simulink model "SysStateMachine"  (R2016b)
settings: Solver=FixedStepAuto  StartTime=0.0  StopTime=inf  RelTol=1e-3
undefined symbols (not defined in the file or in its folder): Chart, nav_statemachine_lib, paramInit
settings Model: Creator=chenjianhui  LastModifiedBy=chenjh43
settings OptimizationCC: MaxStackSize=64
settings DebuggingCC: ParameterTunabilityLossMsg=error
settings HardwareCC: ProdBitPerLong=64  ProdHWDeviceType=Intel->x86-64 (Linux 64)
settings RTWCC: SystemTargetFile=ert.tlc  HardwareBoard=Robot Operating System (ROS)  TLCOptions="-aInlineSetEventsForThisBaseRateFcn=TLC_FALSE -aSuppressMultiTaskScheduler=TLC_FALSE  -aRateBasedStepFcn=0"  TemplateMakefile=ert_default_tmf  Description=Embedded Coder  GenerateReport=on  Toolchain=Catkin  IncludeHyperlinkInReport=on  LaunchReport=on  TargetLang=C++  GenerateTraceInfo=on  GenerateTraceReport=on  GenerateTraceReportSl=on  GenerateTraceReportSf=on  GenerateTraceReportEml=on  GenerateWebview=on
settings CodeAppCC: ForceParamTrailComments=on  IgnoreCustomStorageClasses=off  OperatorAnnotations=on  SimulinkDataObjDesc=on  SFDataObjDesc=on  MATLABFcnDesc=on  InsertBlockDesc=on  MATLABSourceComments=on

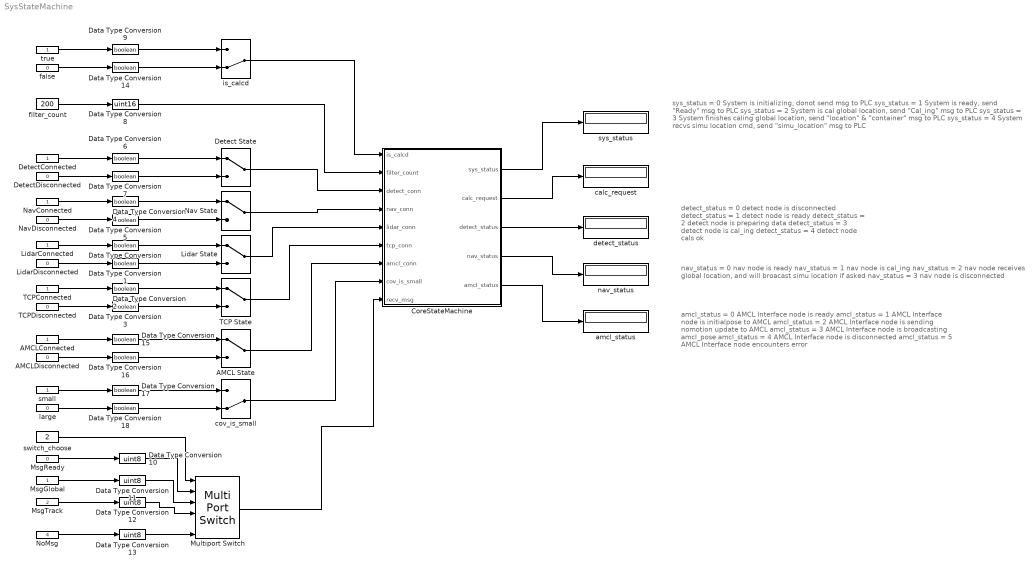
== system SysStateMachine ==
  note: sys_status = 0	System is initializing, donot send msg to PLC
      | sys_status = 1	System is ready, send "Ready" msg to PLC
      | sys_status = 2	System is cal global location, send "Cal_ing" msg to PLC
      | sys_status = 3	System finishes caling global location, send "location" & "container" msg to PLC
      | sys_status = 4	System recvs simu location cmd, send "simu_location" msg to PLC
  note: nav_status = 0 		nav node is ready
      | nav_status = 1 		nav node is cal_ing
      | nav_status = 2 		nav node receives global location, and will broacast simu location if asked
      | nav_status = 3		nav node is disconnected
  note: amcl_status = 0 AMCL Interface node is ready
      | amcl_status = 1 AMCL Interface node is initialpose to AMCL
      | amcl_status = 2 AMCL Interface node is sending nomotion update to AMCL
      | amcl_status = 3 AMCL Interface node is broadcasting amcl_pose
      | amcl_status = 4 AMCL Interface node is disconnected
      | amcl_status = 5 AMCL Interface node encounters error
  note: detect_status = 0		detect node is disconnected
      | detect_status = 1 		detect node is ready
      | detect_status = 2		detect node is preparing data
      | detect_status = 3 		detect node is cal_ing
      | detect_status = 4 		detect node cals ok
  AMCL State : ManualSwitch
  AMCLConnected : Constant
  AMCLDisconnected : Constant  Value=0
  CoreStateMachine : Subsystem  InitFcn=paramInit;
  Data Type Conversion{,1..7,9,14..18} (14 alike) : DataTypeConversion  OutDataTypeStr=boolean
  Data Type Conversion{10..13} (4 alike) : DataTypeConversion  OutDataTypeStr=uint8
  Data Type Conversion8 : DataTypeConversion  OutDataTypeStr=uint16
  Detect State : ManualSwitch
  DetectConnected : Constant
  DetectDisconnected : Constant  Value=0
  Lidar State : ManualSwitch
  LidarConnected : Constant
  LidarDisconnected : Constant  Value=0
  MsgGlobal : Constant
  MsgReady : Constant  Value=0
  MsgTrack : Constant  Value=2
  Multiport Switch : MultiPortSwitch  DataPortOrder=Zero-based contiguous  Inputs=5
  Nav State : ManualSwitch
  NavConnected : Constant
  NavDisconnected : Constant  Value=0
  NoMsg : Constant  Value=4
  TCP State : ManualSwitch
  TCPConnected : Constant
  TCPDisconnected : Constant  Value=0
  amcl_status : Display
  calc_request : Display
  cov_is_small : ManualSwitch  CurrentSetting=0
  detect_status : Display
  false : Constant  Value=0
  filter_count : Constant  Value=200
  is_calcd : ManualSwitch  CurrentSetting=0
  large : Constant  Value=0
  nav_status : Display
  small : Constant
  switch_choose : Constant  Value=2
  sys_status : Display
  true : Constant
  wires:
  LidarConnected/1 -> Data Type Conversion/1
  LidarDisconnected/1 -> Data Type Conversion1/1
  TCPConnected/1 -> Data Type Conversion2/1
  TCPDisconnected/1 -> Data Type Conversion3/1
  Data Type Conversion/1 -> Lidar State/1
  Data Type Conversion1/1 -> Lidar State/2
  Data Type Conversion2/1 -> TCP State/1
  Data Type Conversion3/1 -> TCP State/2
  CoreStateMachine/1(sys_status) -> sys_status/1
  CoreStateMachine/2(calc_request) -> calc_request/1
  CoreStateMachine/3(detect_status) -> detect_status/1
  CoreStateMachine/4(nav_status) -> nav_status/1
  MsgGlobal/1 -> Data Type Conversion11/1
  MsgTrack/1 -> Data Type Conversion12/1
  Data Type Conversion11/1 -> Multiport Switch/3
  Data Type Conversion12/1 -> Multiport Switch/4
  Lidar State/1 -> CoreStateMachine/5(lidar_conn)
  TCP State/1 -> CoreStateMachine/6(tcp_conn)
  NavConnected/1 -> Data Type Conversion4/1
  NavDisconnected/1 -> Data Type Conversion5/1
  Data Type Conversion4/1 -> Nav State/1
  Data Type Conversion5/1 -> Nav State/2
  Nav State/1 -> CoreStateMachine/4(nav_conn)
  DetectConnected/1 -> Data Type Conversion6/1
  DetectDisconnected/1 -> Data Type Conversion7/1
  Data Type Conversion6/1 -> Detect State/1
  Data Type Conversion7/1 -> Detect State/2
  Detect State/1 -> CoreStateMachine/3(detect_conn)
  Data Type Conversion8/1 -> CoreStateMachine/2(filter_count)
  filter_count/1 -> Data Type Conversion8/1
  MsgReady/1 -> Data Type Conversion10/1
  NoMsg/1 -> Data Type Conversion13/1
  Data Type Conversion10/1 -> Multiport Switch/2
  true/1 -> Data Type Conversion9/1
  false/1 -> Data Type Conversion14/1
  Data Type Conversion9/1 -> is_calcd/1
  Data Type Conversion14/1 -> is_calcd/2
  is_calcd/1 -> CoreStateMachine/1(is_calcd)
  CoreStateMachine/5(amcl_status) -> amcl_status/1
  switch_choose/1 -> Multiport Switch/1
  Data Type Conversion13/1 -> Multiport Switch/6
  Multiport Switch/1 -> CoreStateMachine/9(recv_msg)
  AMCLDisconnected/1 -> Data Type Conversion16/1
  Data Type Conversion16/1 -> AMCL State/2
  AMCL State/1 -> CoreStateMachine/7(amcl_conn)
  large/1 -> Data Type Conversion18/1
  Data Type Conversion18/1 -> cov_is_small/2
  cov_is_small/1 -> CoreStateMachine/8(cov_is_small)
  Data Type Conversion17/1 -> cov_is_small/1
  small/1 -> Data Type Conversion17/1
  AMCLConnected/1 -> Data Type Conversion15/1
  Data Type Conversion15/1 -> AMCL State/1

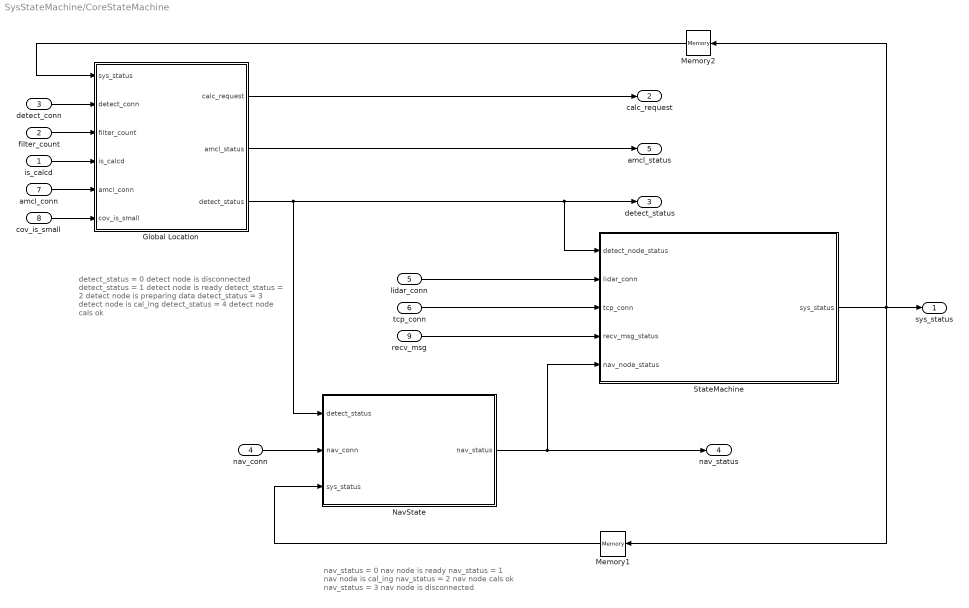
== system SysStateMachine/CoreStateMachine ==
  note: nav_status = 0 		nav node is ready
      | nav_status = 1 		nav node is cal_ing
      | nav_status = 2 		nav node cals ok
      | nav_status = 3		nav node is disconnected
  note: detect_status = 0		detect node is disconnected
      | detect_status = 1 		detect node is ready
      | detect_status = 2		detect node is preparing data
      | detect_status = 3 		detect node is cal_ing
      | detect_status = 4 		detect node cals ok
  is_calcd : Inport
  filter_count : Inport  Port=2
  detect_conn : Inport  Port=3
  nav_conn : Inport  Port=4
  lidar_conn : Inport  Port=5
  tcp_conn : Inport  Port=6
  amcl_conn : Inport  Port=7
  cov_is_small : Inport  Port=8
  recv_msg : Inport  Port=9
  Global Location : Subsystem
  Memory1 : Memory
  Memory2 : Memory
  NavState : Stateflow chart  TreatAsAtomicUnit=on
  StateMachine : Stateflow chart  AncestorBlock=nav_statemachine_lib/Chart  TreatAsAtomicUnit=on
  sys_status : Outport
  calc_request : Outport  Port=2
  detect_status : Outport  Port=3
  nav_status : Outport  Port=4
  amcl_status : Outport  Port=5
  wires:
  NavState/1(nav_status) -> nav_status/1, StateMachine/5(nav_node_status)
  StateMachine/1(sys_status) -> sys_status/1, Memory1/1, Memory2/1
  Memory1/1 -> NavState/3(sys_status)
  recv_msg/1 -> StateMachine/4(recv_msg_status)
  lidar_conn/1 -> StateMachine/2(lidar_conn)
  tcp_conn/1 -> StateMachine/3(tcp_conn)
  nav_conn/1 -> NavState/2(nav_conn)
  Global Location/3(detect_status) -> detect_status/1, StateMachine/1(detect_node_status), NavState/1(detect_status)
  Memory2/1 -> Global Location/1(sys_status)
  detect_conn/1 -> Global Location/2(detect_conn)
  filter_count/1 -> Global Location/3(filter_count)
  is_calcd/1 -> Global Location/4(is_calcd)
  amcl_conn/1 -> Global Location/5(amcl_conn)
  cov_is_small/1 -> Global Location/6(cov_is_small)
  Global Location/1(calc_request) -> calc_request/1
  Global Location/2(amcl_status) -> amcl_status/1

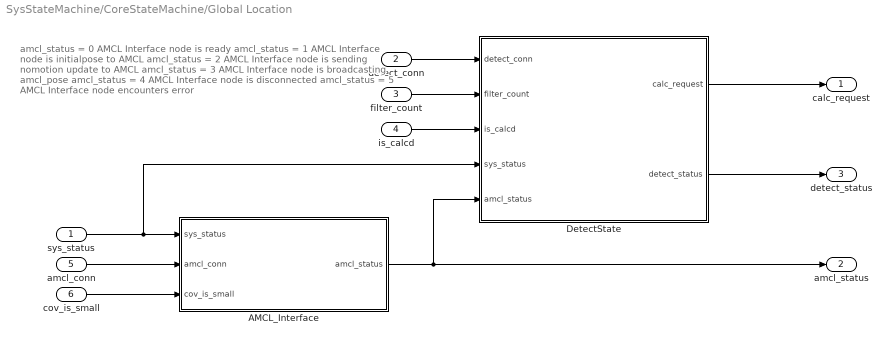
== system SysStateMachine/CoreStateMachine/Global Location ==
  note: amcl_status = 0 AMCL Interface node is ready
      | amcl_status = 1 AMCL Interface node is initialpose to AMCL
      | amcl_status = 2 AMCL Interface node is sending nomotion update to AMCL
      | amcl_status = 3 AMCL Interface node is broadcasting amcl_pose
      | amcl_status = 4 AMCL Interface node is disconnected
      | amcl_status = 5 AMCL Interface node encounters error
  sys_status : Inport
  detect_conn : Inport  Port=2
  filter_count : Inport  Port=3
  is_calcd : Inport  Port=4
  amcl_conn : Inport  Port=5
  cov_is_small : Inport  Port=6
  AMCL_Interface : Stateflow chart  TreatAsAtomicUnit=on
  DetectState : Stateflow chart  TreatAsAtomicUnit=on
  calc_request : Outport
  amcl_status : Outport  Port=2
  detect_status : Outport  Port=3
  wires:
  AMCL_Interface/1(amcl_status) -> amcl_status/1, DetectState/5(amcl_status)
  sys_status/1 -> DetectState/4(sys_status), AMCL_Interface/1(sys_status)
  DetectState/1(calc_request) -> calc_request/1
  DetectState/2(detect_status) -> detect_status/1
  detect_conn/1 -> DetectState/1(detect_conn)
  filter_count/1 -> DetectState/2(filter_count)
  is_calcd/1 -> DetectState/3(is_calcd)
  amcl_conn/1 -> AMCL_Interface/2(amcl_conn)
  cov_is_small/1 -> AMCL_Interface/3(cov_is_small)

== stateflow chart SysStateMachine/CoreStateMachine/StateMachine ==
  settings: updateMethod=DISCRETE  sampleTime=0.01
  state PCReady
    sys_status = 1;
  state Initialization
    sys_status = 0;
  state PLCReady
    sys_status = 1;
  state GlobalLocationOn
    sys_status = 2;
  state GlobalLocationOK
    sys_status = 3;
  state SimuLocation
    sys_status = 4;
  (default) -> Initialization
  Initialization -> PCReady : [lidar_conn == 1 && ...
      | tcp_conn == 1 && ...
      | detect_node_status == 1 && ...
      | nav_node_status == 0]
  SimuLocation -> Initialization [order 1] : [lidar_conn == 0 || ...
      | tcp_conn == 0 || ...
      | detect_node_status == 0 || ...
      | nav_node_status == 3]
  PCReady -> PLCReady [order 2] : [recv_msg_status == 0]
  PCReady -> Initialization [order 1] : [lidar_conn == 0 || ...
      | tcp_conn == 0 || ...
      | detect_node_status == 0 || ...
      | nav_node_status == 3]
  GlobalLocationOK -> Initialization [order 1] : [lidar_conn == 0 || ...
      | tcp_conn == 0 || ...
      | detect_node_status == 0 || ...
      | nav_node_status == 3]
  PLCReady -> Initialization [order 1] : [lidar_conn == 0 || ...
      | tcp_conn == 0 || ...
      | detect_node_status == 0 || ...
      | nav_node_status == 3]
  PLCReady -> GlobalLocationOn [order 2] : [detect_node_status == 1 && ...
      | nav_node_status == 0 && ...
      | recv_msg_status == 1]
  GlobalLocationOn -> Initialization [order 1] : [lidar_conn == 0 || ...
      | tcp_conn == 0 || ...
      | detect_node_status == 0 || ...
      | nav_node_status == 3]
  GlobalLocationOn -> GlobalLocationOK [order 2] : [detect_node_status == 4]
  SimuLocation -> GlobalLocationOn [order 2] : [recv_msg_status == 1]
  GlobalLocationOK -> SimuLocation [order 2] : [nav_node_status == 2 && ...
      | recv_msg_status == 2]
  data: detect_node_status input uint8; lidar_conn input boolean; tcp_conn input boolean; recv_msg_status input uint8; nav_node_status input uint8; sys_status output uint8

== stateflow chart SysStateMachine/CoreStateMachine/NavState ==
  settings: updateMethod=DISCRETE  sampleTime=0.01
  state NavReady
    during:nav_status = 0;
  state NavCalib
    during:nav_status = 1;
  state NavDisconn
    nav_status = 3;
  state NavOK
    during:nav_status = 2;
  NavReady -> NavCalib [order 2] : [sys_status == 2]
  NavCalib -> NavReady [order 2] : [sys_status ~= 2]
  NavCalib -> NavDisconn [order 1] : [nav_conn == 0]
  NavCalib -> NavOK [order 3] : [detect_status == 2]
  NavOK -> NavCalib [order 3] : [sys_status == 2 && ...
      | detect_status != 2]
  NavOK -> NavReady [order 2] : [sys_status == 0 || ...
      | sys_status == 1]
  NavReady -> NavDisconn [order 1] : [nav_conn == 0]
  NavDisconn -> NavReady : [nav_conn == 1]
  (default) -> NavDisconn
  NavOK -> NavDisconn [order 1] : [nav_conn == 0]
  data: detect_status input uint8; nav_conn input boolean; nav_status output uint8; sys_status input uint8

== stateflow chart SysStateMachine/CoreStateMachine/Global Location/DetectState ==
  settings: updateMethod=DISCRETE  sampleTime=0.01
  state DataPreparation
    entry:cal_count = filter_count+counter_times;
    during:detect_status = 2;
  state DetectReady
    during:detect_status = 1;
  state DetectDisconn
    during:detect_status = 0;
  state DetectCal
    entry:calc_request = true;
    during:detect_status = 3;
    exit:calc_request = false;
  state DetectCalOK
    during:detect_status = 4;
  DetectReady -> DataPreparation [order 2] : [sys_status == 2]
  DataPreparation -> DetectReady [order 2] : [sys_status != 2]
  DataPreparation -> DetectDisconn [order 1] : [detect_conn == 0]
  DataPreparation -> DetectCal [order 3] : [filter_count >= cal_count && ...
      | amcl_status == 3]
  DetectCalOK -> DetectReady [order 2] : [sys_status == 3 || ...
      | sys_status == 0 || ...
      | sys_status == 1]
  DetectReady -> DetectDisconn [order 1] : [detect_conn == 0]
  DetectDisconn -> DetectReady : [detect_conn == 1]
  (default) -> DetectDisconn
  DetectCal -> DetectDisconn [order 1] : [detect_conn == 0]
  DetectCalOK -> DetectDisconn [order 1] : [detect_conn == 0]
  DetectCal -> DetectCalOK [order 2] : [is_calcd == true]
  data: detect_conn input boolean; counter_times parameter uint16; cal_count local uint16; filter_count input uint16; calc_request output boolean =false; detect_status output uint8; is_calcd input boolean; sys_status input uint8; amcl_status input uint8

== stateflow chart SysStateMachine/CoreStateMachine/Global Location/AMCL_Interface ==
  settings: updateMethod=DISCRETE  sampleTime=0.01
  state AMCLReady
    during:amcl_status = 0;
  state SendInitPose
    entry:send_count = 0;
    during:amcl_status = 1;
    during:send_count  = send_count + 1;
  state AMCLDisconn
    during:amcl_status = 4;
  state SendToughLocation
    during:amcl_status = 3;
  state UpdatePose
    entry:update_count = 0;
    during:amcl_status = 2;
    during:update_count = update_count + 1;
  state Error
    during:amcl_status = 5;
  AMCLReady -> (junction 20) [order 2] : [sys_status == 2]
  (junction 20) -> SendInitPose : {init_count = 0}
  Error -> AMCLReady
  SendInitPose -> AMCLReady [order 2] : [sys_status != 2]
  SendToughLocation -> AMCLReady [order 2] : [sys_status != 2]
  AMCLReady -> AMCLDisconn [order 1] : [amcl_conn == 0]
  AMCLDisconn -> AMCLReady : [amcl_conn == 1]
  SendInitPose -> AMCLDisconn [order 1] : [amcl_conn == 0]
  UpdatePose -> SendInitPose [order 4] : [cov_is_small == 1]
  SendInitPose -> (junction 24) [order 3] : [send_count >= 3 ]
  (default) -> AMCLDisconn
  UpdatePose -> AMCLDisconn [order 1] : [amcl_conn == 0]
  (junction 24) -> UpdatePose : {init_count = init_count + 1}
  SendToughLocation -> AMCLDisconn [order 1] : [amcl_conn == 0]
  UpdatePose -> SendToughLocation [order 3] : [init_count >= 2 && cov_is_small == 1]
  UpdatePose -> Error [order 2] : [update_count > 200]
  data: sys_status input uint8; amcl_conn input boolean; amcl_status output uint8; cov_is_small input boolean; init_count local uint16; send_count local uint16; update_count local uint16
